simulink model "SingleStreamSSRwithPL"  (R2020a)
settings: Solver=VariableStepAuto  StartTime=0.0  StopTime=inf  RelTol=1e-3
PreLoadFcn:
  | xmcCheckSlxPath(bdroot)
  | SSR4_init
InitFcn:
  | xmcCheckSlxPath(bdroot)
  | SSR4_init;
undefined symbols (not defined in the file): c, FIR_MultiKernel_cin, FIR_MultiKernel_cincout, FIR_MultiKernel_cout, FramesPerVector, S, SHIFT_ACC, SingleStream, T, Taps, ValidDelay, VectorSize, xc7vx485tffg1157
libraries: xbsIndex_r4 x49, ModelComposer x41, simulink x25, dspsrcs4 x1
(part 3 of 3)

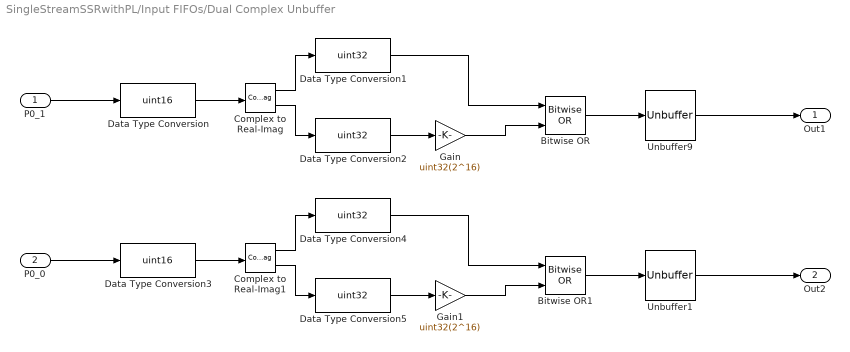
== system SingleStreamSSRwithPL/Input FIFOs/Dual Complex Unbuffer ==
  P0_1 : Inport
  P0_0 : Inport  Port=2
  Bitwise OR : simulink/Logic and Bit Operations/Bitwise Operator  logicop=OR  UseBitMask=off  NumInputPorts=2  BitMask=bin2dec('11011001')  BitMaskRealWorld=Stored Integer
  Bitwise OR1 : simulink/Logic and Bit Operations/Bitwise Operator  logicop=OR  UseBitMask=off  NumInputPorts=2  BitMask=bin2dec('11011001')  BitMaskRealWorld=Stored Integer
  Complex to Real-Imag : ComplexToRealImag
  Complex to Real-Imag1 : ComplexToRealImag
  Data Type Conversion : DataTypeConversion  OutDataTypeStr=uint16  ConvertRealWorld=Stored Integer (SI)
  Data Type Conversion{1..2,4..5} (4 alike) : DataTypeConversion  OutDataTypeStr=uint32  ConvertRealWorld=Stored Integer (SI)
  Data Type Conversion3 : DataTypeConversion  OutDataTypeStr=uint16  ConvertRealWorld=Stored Integer (SI)
  Gain : Gain  Gain=uint32(2^16)  OutDataTypeStr=uint32
  Gain1 : Gain  Gain=uint32(2^16)  OutDataTypeStr=uint32
  Unbuffer1 : Unbuffer
  Unbuffer9 : Unbuffer
  Out1 : Outport
  Out2 : Outport  Port=2
  wires:
  Unbuffer1/1 -> Out2/1
  Unbuffer9/1 -> Out1/1
  Data Type Conversion/1 -> Complex to Real-Imag/1
  P0_1/1 -> Data Type Conversion/1
  Data Type Conversion2/1 -> Gain/1
  Bitwise OR/1 -> Unbuffer9/1
  Complex to Real-Imag/1 -> Data Type Conversion1/1
  Complex to Real-Imag/2 -> Data Type Conversion2/1
  Data Type Conversion1/1 -> Bitwise OR/1
  Gain/1 -> Bitwise OR/2
  Gain1/1 -> Bitwise OR1/2
  Data Type Conversion4/1 -> Bitwise OR1/1
  Complex to Real-Imag1/2 -> Data Type Conversion5/1
  Complex to Real-Imag1/1 -> Data Type Conversion4/1
  Data Type Conversion5/1 -> Gain1/1
  Data Type Conversion3/1 -> Complex to Real-Imag1/1
  P0_0/1 -> Data Type Conversion3/1
  Bitwise OR1/1 -> Unbuffer1/1

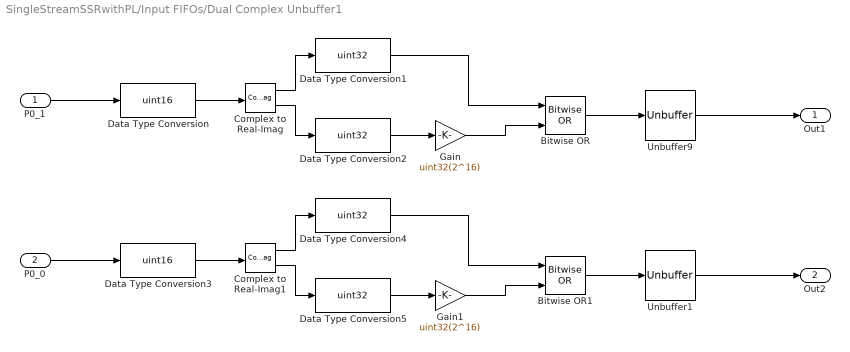
== system SingleStreamSSRwithPL/Input FIFOs/Dual Complex Unbuffer1 ==
  P0_1 : Inport
  P0_0 : Inport  Port=2
  Bitwise OR : simulink/Logic and Bit Operations/Bitwise Operator  logicop=OR  UseBitMask=off  NumInputPorts=2  BitMask=bin2dec('11011001')  BitMaskRealWorld=Stored Integer
  Bitwise OR1 : simulink/Logic and Bit Operations/Bitwise Operator  logicop=OR  UseBitMask=off  NumInputPorts=2  BitMask=bin2dec('11011001')  BitMaskRealWorld=Stored Integer
  Complex to Real-Imag : ComplexToRealImag
  Complex to Real-Imag1 : ComplexToRealImag
  Data Type Conversion : DataTypeConversion  OutDataTypeStr=uint16  ConvertRealWorld=Stored Integer (SI)
  Data Type Conversion{1..2,4..5} (4 alike) : DataTypeConversion  OutDataTypeStr=uint32  ConvertRealWorld=Stored Integer (SI)
  Data Type Conversion3 : DataTypeConversion  OutDataTypeStr=uint16  ConvertRealWorld=Stored Integer (SI)
  Gain : Gain  Gain=uint32(2^16)  OutDataTypeStr=uint32
  Gain1 : Gain  Gain=uint32(2^16)  OutDataTypeStr=uint32
  Unbuffer1 : Unbuffer
  Unbuffer9 : Unbuffer
  Out1 : Outport
  Out2 : Outport  Port=2
  wires:
  Bitwise OR1/1 -> Unbuffer1/1
  P0_0/1 -> Data Type Conversion3/1
  Data Type Conversion3/1 -> Complex to Real-Imag1/1
  Data Type Conversion5/1 -> Gain1/1
  Complex to Real-Imag1/1 -> Data Type Conversion4/1
  Complex to Real-Imag1/2 -> Data Type Conversion5/1
  Data Type Conversion4/1 -> Bitwise OR1/1
  Gain1/1 -> Bitwise OR1/2
  Gain/1 -> Bitwise OR/2
  Data Type Conversion1/1 -> Bitwise OR/1
  Complex to Real-Imag/2 -> Data Type Conversion2/1
  Complex to Real-Imag/1 -> Data Type Conversion1/1
  Bitwise OR/1 -> Unbuffer9/1
  Data Type Conversion2/1 -> Gain/1
  P0_1/1 -> Data Type Conversion/1
  Data Type Conversion/1 -> Complex to Real-Imag/1
  Unbuffer9/1 -> Out1/1
  Unbuffer1/1 -> Out2/1

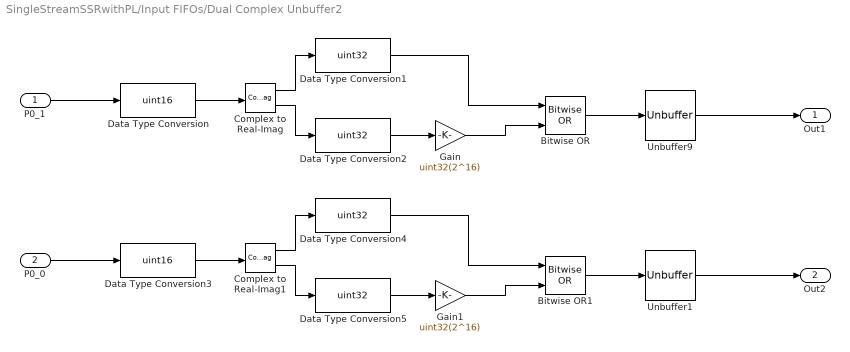
== system SingleStreamSSRwithPL/Input FIFOs/Dual Complex Unbuffer2 ==
  P0_1 : Inport
  P0_0 : Inport  Port=2
  Bitwise OR : simulink/Logic and Bit Operations/Bitwise Operator  logicop=OR  UseBitMask=off  NumInputPorts=2  BitMask=bin2dec('11011001')  BitMaskRealWorld=Stored Integer
  Bitwise OR1 : simulink/Logic and Bit Operations/Bitwise Operator  logicop=OR  UseBitMask=off  NumInputPorts=2  BitMask=bin2dec('11011001')  BitMaskRealWorld=Stored Integer
  Complex to Real-Imag : ComplexToRealImag
  Complex to Real-Imag1 : ComplexToRealImag
  Data Type Conversion : DataTypeConversion  OutDataTypeStr=uint16  ConvertRealWorld=Stored Integer (SI)
  Data Type Conversion{1..2,4..5} (4 alike) : DataTypeConversion  OutDataTypeStr=uint32  ConvertRealWorld=Stored Integer (SI)
  Data Type Conversion3 : DataTypeConversion  OutDataTypeStr=uint16  ConvertRealWorld=Stored Integer (SI)
  Gain : Gain  Gain=uint32(2^16)  OutDataTypeStr=uint32
  Gain1 : Gain  Gain=uint32(2^16)  OutDataTypeStr=uint32
  Unbuffer1 : Unbuffer
  Unbuffer9 : Unbuffer
  Out1 : Outport
  Out2 : Outport  Port=2
  wires:
  Bitwise OR1/1 -> Unbuffer1/1
  P0_0/1 -> Data Type Conversion3/1
  Data Type Conversion3/1 -> Complex to Real-Imag1/1
  Data Type Conversion5/1 -> Gain1/1
  Complex to Real-Imag1/1 -> Data Type Conversion4/1
  Complex to Real-Imag1/2 -> Data Type Conversion5/1
  Data Type Conversion4/1 -> Bitwise OR1/1
  Gain1/1 -> Bitwise OR1/2
  Gain/1 -> Bitwise OR/2
  Data Type Conversion1/1 -> Bitwise OR/1
  Complex to Real-Imag/2 -> Data Type Conversion2/1
  Complex to Real-Imag/1 -> Data Type Conversion1/1
  Bitwise OR/1 -> Unbuffer9/1
  Data Type Conversion2/1 -> Gain/1
  P0_1/1 -> Data Type Conversion/1
  Data Type Conversion/1 -> Complex to Real-Imag/1
  Unbuffer9/1 -> Out1/1
  Unbuffer1/1 -> Out2/1

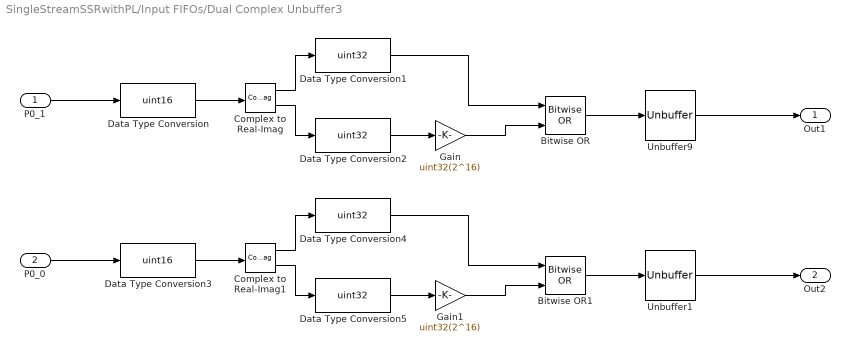
== system SingleStreamSSRwithPL/Input FIFOs/Dual Complex Unbuffer3 ==
  P0_1 : Inport
  P0_0 : Inport  Port=2
  Bitwise OR : simulink/Logic and Bit Operations/Bitwise Operator  logicop=OR  UseBitMask=off  NumInputPorts=2  BitMask=bin2dec('11011001')  BitMaskRealWorld=Stored Integer
  Bitwise OR1 : simulink/Logic and Bit Operations/Bitwise Operator  logicop=OR  UseBitMask=off  NumInputPorts=2  BitMask=bin2dec('11011001')  BitMaskRealWorld=Stored Integer
  Complex to Real-Imag : ComplexToRealImag
  Complex to Real-Imag1 : ComplexToRealImag
  Data Type Conversion : DataTypeConversion  OutDataTypeStr=uint16  ConvertRealWorld=Stored Integer (SI)
  Data Type Conversion{1..2,4..5} (4 alike) : DataTypeConversion  OutDataTypeStr=uint32  ConvertRealWorld=Stored Integer (SI)
  Data Type Conversion3 : DataTypeConversion  OutDataTypeStr=uint16  ConvertRealWorld=Stored Integer (SI)
  Gain : Gain  Gain=uint32(2^16)  OutDataTypeStr=uint32
  Gain1 : Gain  Gain=uint32(2^16)  OutDataTypeStr=uint32
  Unbuffer1 : Unbuffer
  Unbuffer9 : Unbuffer
  Out1 : Outport
  Out2 : Outport  Port=2
  wires:
  Bitwise OR1/1 -> Unbuffer1/1
  P0_0/1 -> Data Type Conversion3/1
  Data Type Conversion3/1 -> Complex to Real-Imag1/1
  Data Type Conversion5/1 -> Gain1/1
  Complex to Real-Imag1/1 -> Data Type Conversion4/1
  Complex to Real-Imag1/2 -> Data Type Conversion5/1
  Data Type Conversion4/1 -> Bitwise OR1/1
  Gain1/1 -> Bitwise OR1/2
  Gain/1 -> Bitwise OR/2
  Data Type Conversion1/1 -> Bitwise OR/1
  Complex to Real-Imag/2 -> Data Type Conversion2/1
  Complex to Real-Imag/1 -> Data Type Conversion1/1
  Bitwise OR/1 -> Unbuffer9/1
  Data Type Conversion2/1 -> Gain/1
  P0_1/1 -> Data Type Conversion/1
  Data Type Conversion/1 -> Complex to Real-Imag/1
  Unbuffer9/1 -> Out1/1
  Unbuffer1/1 -> Out2/1

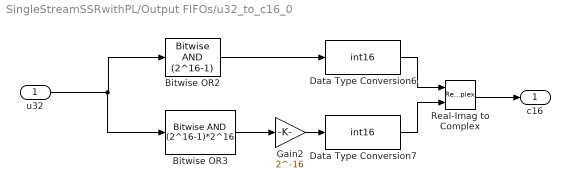
== system SingleStreamSSRwithPL/Output FIFOs/u32_to_c16_0 ==
  u32 : Inport
  Bitwise OR2 : simulink/Logic and Bit Operations/Bitwise Operator  logicop=AND  UseBitMask=on  BitMask=(2^16-1)  BitMaskRealWorld=Stored Integer
  Bitwise OR3 : simulink/Logic and Bit Operations/Bitwise Operator  logicop=AND  UseBitMask=on  BitMask=(2^16-1)*2^16  BitMaskRealWorld=Stored Integer
  Data Type Conversion6 : DataTypeConversion  OutDataTypeStr=int16  ConvertRealWorld=Stored Integer (SI)
  Data Type Conversion7 : DataTypeConversion  OutDataTypeStr=int16  ConvertRealWorld=Stored Integer (SI)
  Gain2 : Gain  Gain=2^-16  OutDataTypeStr=uint32
  Real-Imag to Complex : RealImagToComplex
  c16 : Outport
  wires:
  u32/1 -> Bitwise OR3/1, Bitwise OR2/1
  Gain2/1 -> Data Type Conversion7/1
  Bitwise OR2/1 -> Data Type Conversion6/1
  Data Type Conversion6/1 -> Real-Imag to Complex/1
  Real-Imag to Complex/1 -> c16/1
  Bitwise OR3/1 -> Gain2/1
  Data Type Conversion7/1 -> Real-Imag to Complex/2

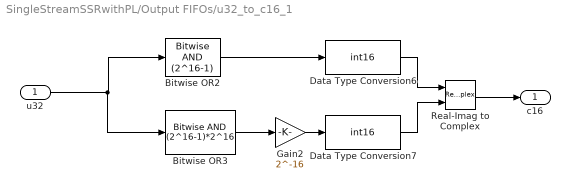
== system SingleStreamSSRwithPL/Output FIFOs/u32_to_c16_1 ==
  u32 : Inport
  Bitwise OR2 : simulink/Logic and Bit Operations/Bitwise Operator  logicop=AND  UseBitMask=on  BitMask=(2^16-1)  BitMaskRealWorld=Stored Integer
  Bitwise OR3 : simulink/Logic and Bit Operations/Bitwise Operator  logicop=AND  UseBitMask=on  BitMask=(2^16-1)*2^16  BitMaskRealWorld=Stored Integer
  Data Type Conversion6 : DataTypeConversion  OutDataTypeStr=int16  ConvertRealWorld=Stored Integer (SI)
  Data Type Conversion7 : DataTypeConversion  OutDataTypeStr=int16  ConvertRealWorld=Stored Integer (SI)
  Gain2 : Gain  Gain=2^-16  OutDataTypeStr=uint32
  Real-Imag to Complex : RealImagToComplex
  c16 : Outport
  wires:
  Data Type Conversion7/1 -> Real-Imag to Complex/2
  Bitwise OR3/1 -> Gain2/1
  Real-Imag to Complex/1 -> c16/1
  Data Type Conversion6/1 -> Real-Imag to Complex/1
  Bitwise OR2/1 -> Data Type Conversion6/1
  Gain2/1 -> Data Type Conversion7/1
  u32/1 -> Bitwise OR2/1, Bitwise OR3/1

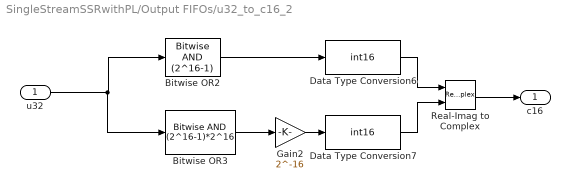
== system SingleStreamSSRwithPL/Output FIFOs/u32_to_c16_2 ==
  u32 : Inport
  Bitwise OR2 : simulink/Logic and Bit Operations/Bitwise Operator  logicop=AND  UseBitMask=on  BitMask=(2^16-1)  BitMaskRealWorld=Stored Integer
  Bitwise OR3 : simulink/Logic and Bit Operations/Bitwise Operator  logicop=AND  UseBitMask=on  BitMask=(2^16-1)*2^16  BitMaskRealWorld=Stored Integer
  Data Type Conversion6 : DataTypeConversion  OutDataTypeStr=int16  ConvertRealWorld=Stored Integer (SI)
  Data Type Conversion7 : DataTypeConversion  OutDataTypeStr=int16  ConvertRealWorld=Stored Integer (SI)
  Gain2 : Gain  Gain=2^-16  OutDataTypeStr=uint32
  Real-Imag to Complex : RealImagToComplex
  c16 : Outport
  wires:
  u32/1 -> Bitwise OR3/1, Bitwise OR2/1
  Gain2/1 -> Data Type Conversion7/1
  Bitwise OR2/1 -> Data Type Conversion6/1
  Data Type Conversion6/1 -> Real-Imag to Complex/1
  Real-Imag to Complex/1 -> c16/1
  Bitwise OR3/1 -> Gain2/1
  Data Type Conversion7/1 -> Real-Imag to Complex/2

== system SingleStreamSSRwithPL/Output FIFOs/u32_to_c16_3 ==
  u32 : Inport
  Bitwise OR2 : simulink/Logic and Bit Operations/Bitwise Operator  logicop=AND  UseBitMask=on  BitMask=(2^16-1)  BitMaskRealWorld=Stored Integer
  Bitwise OR3 : simulink/Logic and Bit Operations/Bitwise Operator  logicop=AND  UseBitMask=on  BitMask=(2^16-1)*2^16  BitMaskRealWorld=Stored Integer
  Data Type Conversion6 : DataTypeConversion  OutDataTypeStr=int16  ConvertRealWorld=Stored Integer (SI)
  Data Type Conversion7 : DataTypeConversion  OutDataTypeStr=int16  ConvertRealWorld=Stored Integer (SI)
  Gain2 : Gain  Gain=2^-16  OutDataTypeStr=uint32
  Real-Imag to Complex : RealImagToComplex
  c16 : Outport
  wires:
  Data Type Conversion7/1 -> Real-Imag to Complex/2
  Bitwise OR3/1 -> Gain2/1
  Real-Imag to Complex/1 -> c16/1
  Data Type Conversion6/1 -> Real-Imag to Complex/1
  Bitwise OR2/1 -> Data Type Conversion6/1
  Gain2/1 -> Data Type Conversion7/1
  u32/1 -> Bitwise OR2/1, Bitwise OR3/1

== system SingleStreamSSRwithPL/Output FIFOs/u32_to_c16_4 ==
  u32 : Inport
  Bitwise OR2 : simulink/Logic and Bit Operations/Bitwise Operator  logicop=AND  UseBitMask=on  BitMask=(2^16-1)  BitMaskRealWorld=Stored Integer
  Bitwise OR3 : simulink/Logic and Bit Operations/Bitwise Operator  logicop=AND  UseBitMask=on  BitMask=(2^16-1)*2^16  BitMaskRealWorld=Stored Integer
  Data Type Conversion6 : DataTypeConversion  OutDataTypeStr=int16  ConvertRealWorld=Stored Integer (SI)
  Data Type Conversion7 : DataTypeConversion  OutDataTypeStr=int16  ConvertRealWorld=Stored Integer (SI)
  Gain2 : Gain  Gain=2^-16  OutDataTypeStr=uint32
  Real-Imag to Complex : RealImagToComplex
  c16 : Outport
  wires:
  u32/1 -> Bitwise OR3/1, Bitwise OR2/1
  Gain2/1 -> Data Type Conversion7/1
  Bitwise OR2/1 -> Data Type Conversion6/1
  Data Type Conversion6/1 -> Real-Imag to Complex/1
  Real-Imag to Complex/1 -> c16/1
  Bitwise OR3/1 -> Gain2/1
  Data Type Conversion7/1 -> Real-Imag to Complex/2

== system SingleStreamSSRwithPL/Output FIFOs/u32_to_c16_5 ==
  u32 : Inport
  Bitwise OR2 : simulink/Logic and Bit Operations/Bitwise Operator  logicop=AND  UseBitMask=on  BitMask=(2^16-1)  BitMaskRealWorld=Stored Integer
  Bitwise OR3 : simulink/Logic and Bit Operations/Bitwise Operator  logicop=AND  UseBitMask=on  BitMask=(2^16-1)*2^16  BitMaskRealWorld=Stored Integer
  Data Type Conversion6 : DataTypeConversion  OutDataTypeStr=int16  ConvertRealWorld=Stored Integer (SI)
  Data Type Conversion7 : DataTypeConversion  OutDataTypeStr=int16  ConvertRealWorld=Stored Integer (SI)
  Gain2 : Gain  Gain=2^-16  OutDataTypeStr=uint32
  Real-Imag to Complex : RealImagToComplex
  c16 : Outport
  wires:
  Data Type Conversion7/1 -> Real-Imag to Complex/2
  Bitwise OR3/1 -> Gain2/1
  Real-Imag to Complex/1 -> c16/1
  Data Type Conversion6/1 -> Real-Imag to Complex/1
  Bitwise OR2/1 -> Data Type Conversion6/1
  Gain2/1 -> Data Type Conversion7/1
  u32/1 -> Bitwise OR2/1, Bitwise OR3/1

== system SingleStreamSSRwithPL/Output FIFOs/u32_to_c16_6 ==
  u32 : Inport
  Bitwise OR2 : simulink/Logic and Bit Operations/Bitwise Operator  logicop=AND  UseBitMask=on  BitMask=(2^16-1)  BitMaskRealWorld=Stored Integer
  Bitwise OR3 : simulink/Logic and Bit Operations/Bitwise Operator  logicop=AND  UseBitMask=on  BitMask=(2^16-1)*2^16  BitMaskRealWorld=Stored Integer
  Data Type Conversion6 : DataTypeConversion  OutDataTypeStr=int16  ConvertRealWorld=Stored Integer (SI)
  Data Type Conversion7 : DataTypeConversion  OutDataTypeStr=int16  ConvertRealWorld=Stored Integer (SI)
  Gain2 : Gain  Gain=2^-16  OutDataTypeStr=uint32
  Real-Imag to Complex : RealImagToComplex
  c16 : Outport
  wires:
  u32/1 -> Bitwise OR3/1, Bitwise OR2/1
  Gain2/1 -> Data Type Conversion7/1
  Bitwise OR2/1 -> Data Type Conversion6/1
  Data Type Conversion6/1 -> Real-Imag to Complex/1
  Real-Imag to Complex/1 -> c16/1
  Bitwise OR3/1 -> Gain2/1
  Data Type Conversion7/1 -> Real-Imag to Complex/2

== system SingleStreamSSRwithPL/Output FIFOs/u32_to_c16_7 ==
  u32 : Inport
  Bitwise OR2 : simulink/Logic and Bit Operations/Bitwise Operator  logicop=AND  UseBitMask=on  BitMask=(2^16-1)  BitMaskRealWorld=Stored Integer
  Bitwise OR3 : simulink/Logic and Bit Operations/Bitwise Operator  logicop=AND  UseBitMask=on  BitMask=(2^16-1)*2^16  BitMaskRealWorld=Stored Integer
  Data Type Conversion6 : DataTypeConversion  OutDataTypeStr=int16  ConvertRealWorld=Stored Integer (SI)
  Data Type Conversion7 : DataTypeConversion  OutDataTypeStr=int16  ConvertRealWorld=Stored Integer (SI)
  Gain2 : Gain  Gain=2^-16  OutDataTypeStr=uint32
  Real-Imag to Complex : RealImagToComplex
  c16 : Outport
  wires:
  Data Type Conversion7/1 -> Real-Imag to Complex/2
  Bitwise OR3/1 -> Gain2/1
  Real-Imag to Complex/1 -> c16/1
  Data Type Conversion6/1 -> Real-Imag to Complex/1
  Bitwise OR2/1 -> Data Type Conversion6/1
  Gain2/1 -> Data Type Conversion7/1
  u32/1 -> Bitwise OR2/1, Bitwise OR3/1

== matlab function SingleStreamSSRwithPL/ComplexSource4/MATLAB Function ==
  data: u input; y1 output; y2 output; y3 output; y4 output; y5 output; y6 output; y7 output; y8 output; valid output; v input
function [y1,y2,y3,y4,y5,y6,y7,y8,valid] = fcn(u,v)


y1 = u(1:8:end);
y2 = u(2:8:end);
y3 = u(3:8:end);
y4 = u(4:8:end);
y5 = u(5:8:end);
y6 = u(6:8:end);
y7 = u(7:8:end);
y8 = u(8:8:end);

valid = v;
